simulink model "aa2"  (R2024b)
settings: Solver=FixedStepAuto  StartTime=0.0  StopTime=0.5  MaxStep=1e-6  RelTol=1e-3
libraries: spsIGBTDiodeLib x6, spsOffDelayLib x3, spsOnDelayLib x3, spsThreePhaseSeriesRLCBranchLib x3, simulink x2, spsDCVoltageSourceLib x1, spsGroundLib x1, spsThreePhaseVIMeasurementLib x1, sps_lib x1
settings Model: Creator=Cybor  LastModifiedBy=86195

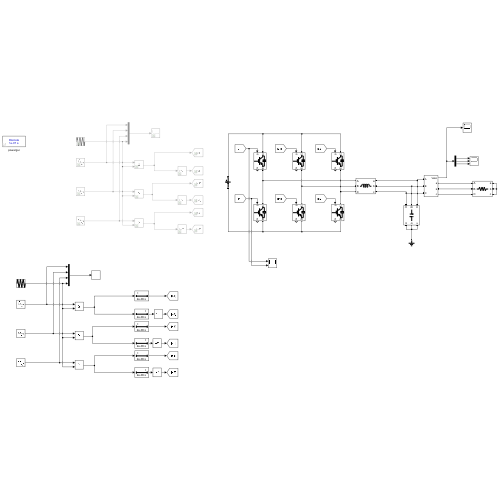
[thumbnail: Simulink's stored preview of the top-level diagram]
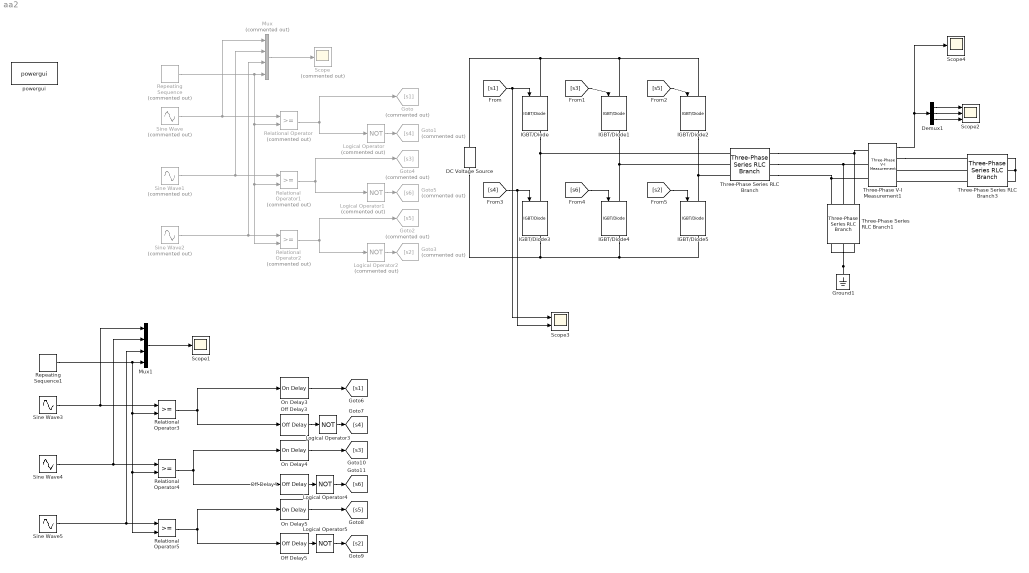
== system aa2 ==
  DC Voltage Source : spsDCVoltageSourceLib/DC Voltage Source  Amplitude=100  Measurements=None
  Demux1 : Demux  Outputs=3
  Goto : Goto  Commented=on  GotoTag=s1
  Goto1 : Goto  Commented=on  GotoTag=s4
  Goto2 : Goto  Commented=on  GotoTag=s5
  Goto3 : Goto  Commented=on  GotoTag=s2
  Goto4 : Goto  Commented=on  GotoTag=s3
  Goto5 : Goto  Commented=on  GotoTag=s6
  Ground1 : spsGroundLib/Ground  LConnTagsString=a
  IGBT/Diode{,1..5} (6 alike) : spsIGBTDiodeLib/IGBT//Diode  Ron=1e-3  Rs=1e5  Cs=inf  Measurements=on
  Logical Operator : Logic  Commented=on  Operator=NOT  AllPortsSameDT=off  OutDataTypeStr=boolean
  Logical Operator1 : Logic  Commented=on  Operator=NOT  AllPortsSameDT=off  OutDataTypeStr=boolean
  Logical Operator2 : Logic  Commented=on  Operator=NOT  AllPortsSameDT=off  OutDataTypeStr=boolean
  Logical Operator3 : Logic  Operator=NOT  AllPortsSameDT=off  OutDataTypeStr=boolean
  Logical Operator4 : Logic  Operator=NOT  AllPortsSameDT=off  OutDataTypeStr=boolean
  Logical Operator5 : Logic  Operator=NOT  AllPortsSameDT=off  OutDataTypeStr=boolean
  Mux : Mux  Commented=on
  Mux1 : Mux
  Off Delay3 : spsOffDelayLib/Off Delay  DelayType=Off delay  delay=2e-6  ic=1  Ts=0
      settings: LibrarySourceBlock=sps_lib/Control/Off Delay
  Off Delay4 : spsOffDelayLib/Off Delay  DelayType=Off delay  delay=2e-6  ic=1  Ts=0
      settings: LibrarySourceBlock=sps_lib/Control/Off Delay
  Off Delay5 : spsOffDelayLib/Off Delay  DelayType=Off delay  delay=2e-6  ic=1  Ts=0
      settings: LibrarySourceBlock=sps_lib/Control/Off Delay
  On Delay3 : spsOnDelayLib/On Delay  DelayType=On delay  delay=2e-6  ic=0  Ts=0
  On Delay4 : spsOnDelayLib/On Delay  DelayType=On delay  delay=2e-6  ic=0  Ts=0
  On Delay5 : spsOnDelayLib/On Delay  DelayType=On delay  delay=2e-6  ic=0  Ts=0
  Relational Operator : RelationalOperator  Commented=on  OutDataTypeStr=boolean  RndMeth=Simplest  InputSameDT=off
  Relational Operator1 : RelationalOperator  Commented=on  OutDataTypeStr=boolean  RndMeth=Simplest  InputSameDT=off
  Relational Operator2 : RelationalOperator  Commented=on  OutDataTypeStr=boolean  RndMeth=Simplest  InputSameDT=off
  Relational Operator3 : RelationalOperator  OutDataTypeStr=boolean  RndMeth=Simplest  InputSameDT=off
  Relational Operator4 : RelationalOperator  OutDataTypeStr=boolean  RndMeth=Simplest  InputSameDT=off
  Relational Operator5 : RelationalOperator  OutDataTypeStr=boolean  RndMeth=Simplest  InputSameDT=off
  Repeating Sequence : simulink/Sources/Repeating Sequence  Commented=on  rep_seq_t=[0 1 3 4]*1/6000  rep_seq_y=[0 1 -1 0]
  Repeating Sequence1 : simulink/Sources/Repeating Sequence  rep_seq_t=[0 1 3 4]*1/6000  rep_seq_y=[0 1 -1 0]
  Scope : Scope  Commented=on
  Scope1 : Scope
  Scope2 : Scope  NumInputPorts=3
  Scope3 : Scope  NumInputPorts=2
  Scope4 : Scope
  Sine Wave : Sin  Commented=on  Amplitude=0.9  Frequency=2*pi*50  SampleTime=0
  Sine Wave1 : Sin  Commented=on  Amplitude=0.9  Frequency=2*pi*50  Phase=2*pi/3  SampleTime=0
  Sine Wave2 : Sin  Commented=on  Amplitude=0.9  Frequency=2*pi*50  Phase=-2*pi/3  SampleTime=0
  Sine Wave3 : Sin  Amplitude=0.9  Frequency=2*pi*50  SampleTime=0
  Sine Wave4 : Sin  Amplitude=0.9  Frequency=2*pi*50  Phase=2*pi/3  SampleTime=0
  Sine Wave5 : Sin  Amplitude=0.9  Frequency=2*pi*50  Phase=-2*pi/3  SampleTime=0
  Three-Phase Series RLC Branch : spsThreePhaseSeriesRLCBranchLib/Three-Phase Series RLC Branch  LConnTagsString=A|B|C  RConnTagsString=A|B|C  BranchType=L  Resistance=1  Inductance=5e-3  Capacitance=1e-6  Measurements=None
  Three-Phase Series RLC Branch1 : spsThreePhaseSeriesRLCBranchLib/Three-Phase Series RLC Branch  LConnTagsString=A|B|C  RConnTagsString=A|B|C  BranchType=C  Resistance=1  Inductance=1e-3  Capacitance=2.2e-6  Measurements=None
  Three-Phase Series RLC Branch3 : spsThreePhaseSeriesRLCBranchLib/Three-Phase Series RLC Branch  LConnTagsString=A|B|C  RConnTagsString=A|B|C  BranchType=R  Resistance=10  Inductance=2e-6  Capacitance=1e-6  Measurements=None
  Three-Phase V-I Measurement1 : spsThreePhaseVIMeasurementLib/Three-Phase V-I Measurement  VoltageMeasurement=phase-to-ground  SetLabelV=off  LabelV=Vabc  Vpu=off  VpuLL=off  CurrentMeasurement=no  SetLabelI=off  LabelI=Iabc  Ipu=off  Pbase=100e6  Vbase=500e3  OutputType=Complex  PhasorSimulation=off  PSBequivalent=0
  powergui : sps_lib/powergui  Priority=1  SimulationMode=Discrete  SampleTime=1e-7  frequency=60  Iterations=50  frequencyindice=0  Pbase=100e6  ErrMax=1e-4  UnitsV=kV  UnitsW=MW  buscounter=0  FunctionMessages=off  echomessages=off  EnableUseOfTLC=off  CurrentSourceSwitches=off  DisableSnubberDevices=off  DisableRonSwitches=off  DisableVfSwitches=off  DisplayEquations=off  AutomaticDiscreteSolvers=off  SolverType=Tustin/Backward Euler (TBE)  Interpol=off  ExternalGateDelay=off  methode=off  Ts=100  x0status=blocks  SPID=on  SwTol=0  HookPort=off  NonlinearTolerance=1e-4  nMaxIteration=100  ContinueOnMaxIteration=off  RestoreLinks=warning  ResistiveCurrentMeasurement=off  Frange=[0:2:500]  Ylog=off  Xlog=on  ShowGrid=off  save=off  variable=ZData  structure=0  ZoomFFT=off  StartTime=0.0  cycles=1  DisplayStyle=1  fundamental=60  FreqAxis=off  MaxFrequency=1000  frequencyindicesteady=1  RmsSteady=1  display=off
  wires:
  Mux/1 -> Scope/1
  Repeating Sequence/1 -> Relational Operator1/2, Relational Operator2/2, Relational Operator/2, Mux/4
  Sine Wave/1 -> Relational Operator/1, Mux/1
  Sine Wave1/1 -> Relational Operator1/1, Mux/2
  Sine Wave2/1 -> Relational Operator2/1, Mux/3
  Logical Operator/1 -> Goto1/1
  Logical Operator1/1 -> Goto5/1
  Logical Operator2/1 -> Goto3/1
  [s1] -> Scope3/1, IGBT/Diode/1
  [s3] -> IGBT/Diode1/1
  [s5] -> IGBT/Diode2/1
  [s4] -> IGBT/Diode3/1, Scope3/2
  [s6] -> IGBT/Diode4/1
  [s2] -> IGBT/Diode5/1
  Demux1/3 -> Scope2/3
  Demux1/2 -> Scope2/2
  Three-Phase V-I Measurement1/1 -> Scope4/1, Demux1/1
  Demux1/1 -> Scope2/1
  Relational Operator/1 -> Logical Operator/1, Goto/1
  Relational Operator1/1 -> Logical Operator1/1, Goto4/1
  Relational Operator2/1 -> Goto2/1, Logical Operator2/1
  Off Delay4/1 -> Logical Operator4/1
  Off Delay5/1 -> Logical Operator5/1
  Off Delay3/1 -> Logical Operator3/1
  On Delay5/1 -> [s5]
  On Delay3/1 -> [s1]
  Logical Operator4/1 -> [s6]
  On Delay4/1 -> [s3]
  Logical Operator3/1 -> [s4]
  Logical Operator5/1 -> [s2]
  Relational Operator3/1 -> Off Delay3/1, On Delay3/1
  Sine Wave3/1 -> Relational Operator3/1, Mux1/1
  Repeating Sequence1/1 -> Relational Operator4/2, Relational Operator5/2, Relational Operator3/2, Mux1/4
  Relational Operator5/1 -> Off Delay5/1, On Delay5/1
  Mux1/1 -> Scope1/1
  Sine Wave4/1 -> Relational Operator4/1, Mux1/2
  Relational Operator4/1 -> Off Delay4/1, On Delay4/1
  Sine Wave5/1 -> Relational Operator5/1, Mux1/3
  connections:
  DC Voltage Source/RConn1 -- IGBT/Diode/LConn1 -- IGBT/Diode1/LConn1 -- IGBT/Diode2/LConn1
  IGBT/Diode/RConn1 -- Three-Phase Series RLC Branch/LConn1 -- IGBT/Diode3/LConn1
  IGBT/Diode1/RConn1 -- Three-Phase Series RLC Branch/LConn2 -- IGBT/Diode4/LConn1
  IGBT/Diode2/RConn1 -- Three-Phase Series RLC Branch/LConn3 -- IGBT/Diode5/LConn1
  DC Voltage Source/LConn1 -- IGBT/Diode3/RConn1 -- IGBT/Diode4/RConn1 -- IGBT/Diode5/RConn1
  Ground1/LConn1 -- Three-Phase Series RLC Branch1/RConn3 -- Three-Phase Series RLC Branch1/RConn1 -- Three-Phase Series RLC Branch1/RConn2
  Three-Phase Series RLC Branch/RConn2 -- Three-Phase V-I Measurement1/LConn2 -- Three-Phase Series RLC Branch1/LConn2
  Three-Phase Series RLC Branch/RConn1 -- Three-Phase Series RLC Branch1/LConn3 -- Three-Phase V-I Measurement1/LConn1
  Three-Phase Series RLC Branch3/RConn1 -- Three-Phase Series RLC Branch3/RConn2 -- Three-Phase Series RLC Branch3/RConn3
  Three-Phase Series RLC Branch/RConn3 -- Three-Phase V-I Measurement1/LConn3 -- Three-Phase Series RLC Branch1/LConn1
  Three-Phase Series RLC Branch3/LConn3 -- Three-Phase V-I Measurement1/RConn3
  Three-Phase Series RLC Branch3/LConn2 -- Three-Phase V-I Measurement1/RConn2
  Three-Phase V-I Measurement1/RConn1 -- Three-Phase Series RLC Branch3/LConn1
